simulink model "Pole_placement_down"  (R2023b)
settings: Solver=VariableStepAuto  StartTime=0.0  StopTime=20.0  RelTol=1e-3
values from neighbouring files (symbols this model uses):
  A = double(A)    [consistent.m]    (also in dyn_model_mark.m)
  B = double(B)    [consistent.m]    (also in dyn_model_mark.m)
  x1_bar = 0    [consistent.m]    (also in dyn_model_mark.m)
  x3_bar = 0    [consistent.m]    (also in dyn_model_mark.m = 3.14159265359)
undefined symbols (not defined in the file or in its folder): K_pp
libraries: simulink_extras x3
settings Model: Creator=Mark  LastModifiedBy=Mark

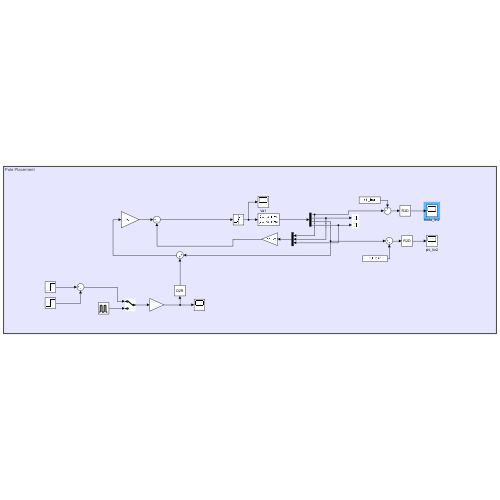
[thumbnail: Simulink's stored preview of the top-level diagram]
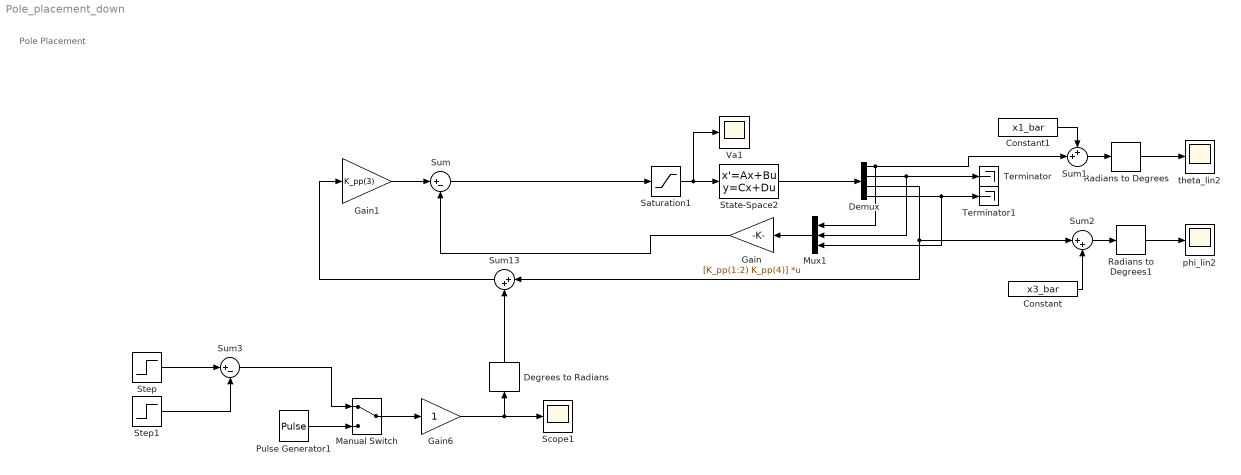
== system Pole_placement_down ==
  note: Pole Placement
  Constant : Constant  Value=x3_bar
  Constant1 : Constant  Value=x1_bar
  Degrees to Radians : simulink_extras/Transformations/Degrees to Radians
  Demux : Demux
  Gain : Gain  Gain=[K_pp(1:2) K_pp(4)]  Multiplication=Matrix(K*u) (u vector)
  Gain1 : Gain  Gain=K_pp(3)
  Gain6 : Gain
  Manual Switch : ManualSwitch
  Mux1 : Mux  Inputs=3
  Pulse Generator1 : DiscretePulseGenerator  PulseType=Time based  Period=10000  PulseWidth=0.005  PhaseDelay=30
  Radians to Degrees : simulink_extras/Transformations/Radians to Degrees
  Radians to Degrees1 : simulink_extras/Transformations/Radians to Degrees
  Saturation1 : Saturate  UpperLimit=10  LowerLimit=-10
  Scope1 : Scope
  State-Space2 : StateSpace  A=A  B=B  C=eye(4)  D=zeros(4,1)  InitialCondition=[0 0 0 0]
  Step : Step  Time=5  SampleTime=0
  Step1 : Step  Time=5.05  SampleTime=0
  Sum : Sum  Inputs=|+-
  Sum1 : Sum  Inputs=++|
  Sum13 : Sum  Inputs=|++
  Sum2 : Sum  Inputs=|++
  Sum3 : Sum  Inputs=|+-
  Terminator : Terminator
  Terminator1 : Terminator
  Va1 : Scope
  phi_lin2 : Scope
  theta_lin2 : Scope
  wires:
  Constant/1 -> Sum2/2
  Mux1/1 -> Gain/1
  State-Space2/1 -> Demux/1
  Constant1/1 -> Sum1/1
  Sum2/1 -> Radians to Degrees1/1
  Sum1/1 -> Radians to Degrees/1
  Degrees to Radians/1 -> Sum13/2
  Demux/4 -> Mux1/3, Terminator1/1
  Sum13/1 -> Gain1/1
  Gain1/1 -> Sum/1
  Radians to Degrees/1 -> theta_lin2/1
  Demux/2 -> Mux1/2, Terminator/1
  Saturation1/1 -> Va1/1, State-Space2/1
  Demux/1 -> Mux1/1, Sum1/2
  Radians to Degrees1/1 -> phi_lin2/1
  Demux/3 -> Sum2/1, Sum13/1
  Gain/1 -> Sum/2
  Sum/1 -> Saturation1/1
  Pulse Generator1/1 -> Manual Switch/2
  Sum3/1 -> Manual Switch/1
  Manual Switch/1 -> Gain6/1
  Step/1 -> Sum3/1
  Gain6/1 -> Scope1/1, Degrees to Radians/1
  Step1/1 -> Sum3/2
